simulink model "RB"  (R2024b)
settings: Solver=ode4  StartTime=0.0  StopTime=T_end_RB  FixedStep=0.01  RelTol=1e-3
values from neighbouring files (symbols this model uses):
  A = ly*lz    (= 0.25)    [Main.m]
  CD = 2.2    [Main.m]
  delta_Vz_RB = (omega_target/4)*delta_x_RB    [Main.m]
  dp0_RB = dpf_HOH    [Main.m]
  Dt = 0.01    [Main.m]
  Dt_con = 0.02    [Main.m]
  Dt_guid = 1    [Main.m]
  kf = 4    [Main.m]
  landa_RB = 1    [Main.m]
  m_c0 = 50    [Main.m]
  omega_target = (mu/r_target^3)^0.5    (= 0.00113136572666)    [Main.m]
  p0_RB = pf_HOH    [Main.m]
  rho = 1*10^(-12)    (= 1e-12)    [Main.m]
  S_RB = 0.5    [Main.m]
  T1_RB = 10    [Main.m]
  T2_RB = T1_RB + T_RB/2    (= 2786.81441073)    [Main.m]
  tau = -ton/(log(1-(Uon-Uoff)/(Tmax*kf)))    [Main.m]
  Total_max_thrust = n*Tmax    (= 2)    [Main.m]
  Uoff = 0.7    [Main.m]
  Uon = 1    [Main.m]
  Vx = omega_target*r_target    (= 7668.56094333)    [Main.m]
settings Model: Creator=corte  LastModifiedBy=aless
settings RTWCC: GPUComputeCapability=3.5

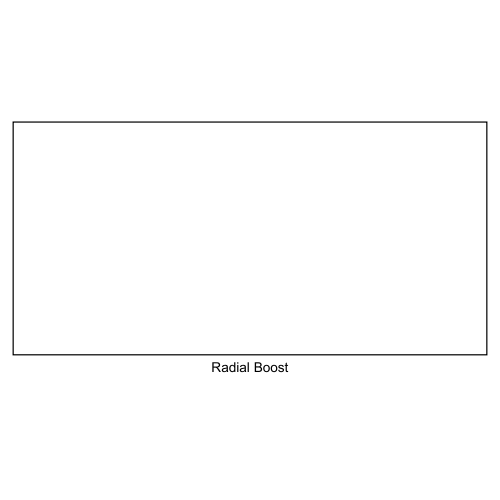
[thumbnail: Simulink's stored preview of the top-level diagram]
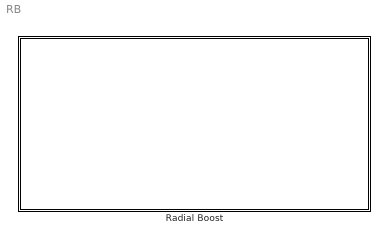
== system RB ==
  Radial Boost : Subsystem

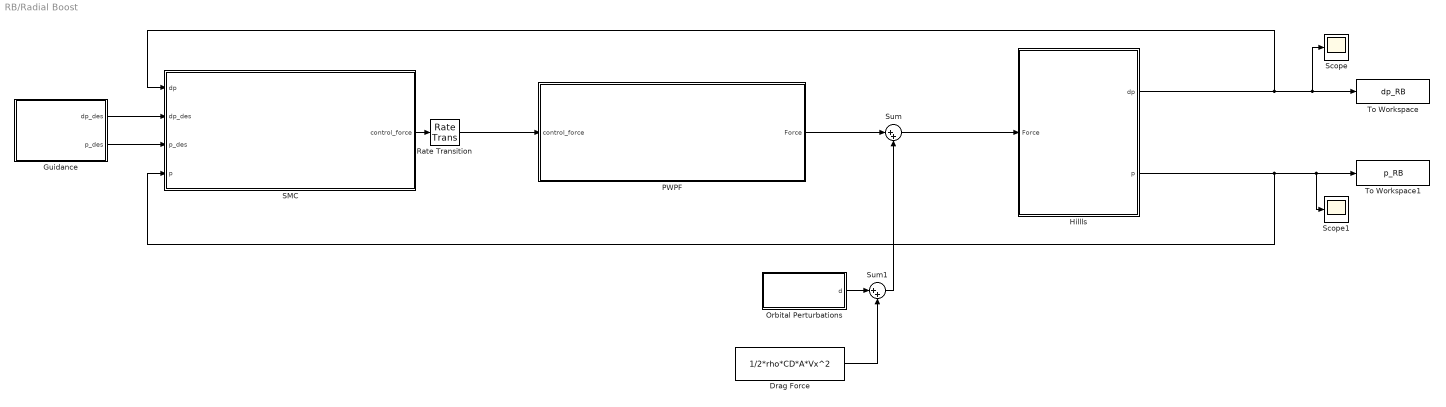
== system RB/Radial Boost ==
  Drag Force : Constant  Value=1/2*rho*CD*A*Vx^2
  Guidance : Subsystem
  Hillls : Subsystem
  Orbital Perturbations : Subsystem
  PWPF : Subsystem
  Rate Transition : RateTransition  InitialCondition=Dt_con  OutPortSampleTime=Dt
  SMC : Subsystem
  Scope : Scope
  Scope1 : Scope
  Sum : Sum  Inputs=|++
  Sum1 : Sum  Inputs=|++
  To Workspace : ToWorkspace  VariableName=dp_RB  SaveFormat=Timeseries  SampleTime=-1
  To Workspace1 : ToWorkspace  VariableName=p_RB  SaveFormat=Timeseries  SampleTime=-1
  wires:
  SMC/1(control_force) -> Rate Transition/1
  Guidance/2(p_des) -> SMC/3(p_des)
  Guidance/1(dp_des) -> SMC/2(dp_des)
  Hillls/2(p) -> Scope1/1, To Workspace1/1, SMC/4(p)
  Hillls/1(dp) -> Scope/1, To Workspace/1, SMC/1(dp)
  Rate Transition/1 -> PWPF/1(control_force)
  Sum1/1 -> Sum/2
  Drag Force/1 -> Sum1/2
  Orbital Perturbations/1(d) -> Sum1/1
  Sum/1 -> Hillls/1(Force)
  PWPF/1(Force) -> Sum/1

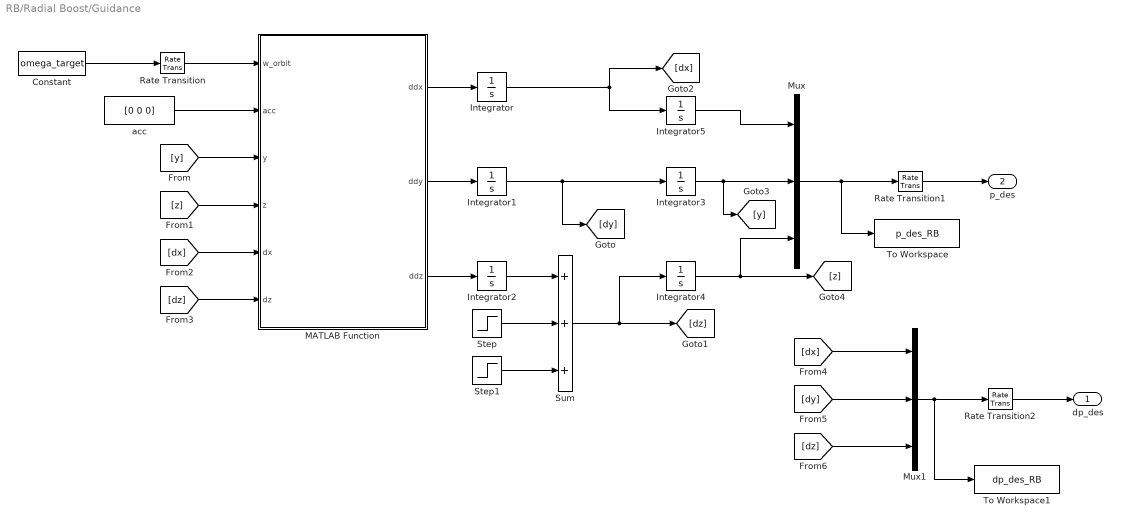
== system RB/Radial Boost/Guidance ==
  Constant : Constant  Value=omega_target
  Integrator : Integrator  InitialCondition=dp0_RB(1)
  Integrator1 : Integrator  InitialCondition=dp0_RB(2)
  Integrator2 : Integrator  InitialCondition=dp0_RB(3)
  Integrator3 : Integrator  InitialCondition=p0_RB(2)
  Integrator4 : Integrator  InitialCondition=p0_RB(3)
  Integrator5 : Integrator  InitialCondition=p0_RB(1)
  MATLAB Function : MATLAB Function  TreatAsAtomicUnit=on
  Mux : Mux  Inputs=3
  Mux1 : Mux  Inputs=3
  Rate Transition : RateTransition  InitialCondition=Dt  OutPortSampleTime=Dt_guid
  Rate Transition1 : RateTransition  InitialCondition=Dt_guid  OutPortSampleTime=Dt
  Rate Transition2 : RateTransition  InitialCondition=Dt_guid  OutPortSampleTime=Dt
  Step : Step  Time=T1_RB  After=delta_Vz_RB  SampleTime=0
  Step1 : Step  Time=T2_RB  After=delta_Vz_RB  SampleTime=0
  Sum : Sum  Inputs=+++
  To Workspace : ToWorkspace  VariableName=p_des_RB  SaveFormat=Timeseries  SampleTime=-1
  To Workspace1 : ToWorkspace  VariableName=dp_des_RB  SaveFormat=Timeseries  SampleTime=-1
  acc : Constant  Value=[0 0 0]
  dp_des : Outport
  p_des : Outport  Port=2
  wires:
  Integrator/1 -> Integrator5/1, [dx]
  Mux/1 -> Rate Transition1/1, To Workspace/1
  Integrator3/1 -> [y], Mux/2
  Integrator4/1 -> [z], Mux/3
  [y] -> MATLAB Function/3(y)
  [dx] -> Mux1/1
  [dz] -> Mux1/3
  acc/1 -> MATLAB Function/2(acc)
  MATLAB Function/1(ddx) -> Integrator/1
  Mux1/1 -> To Workspace1/1, Rate Transition2/1
  [dy] -> Mux1/2
  [dx] -> MATLAB Function/5(dx)
  [z] -> MATLAB Function/4(z)
  Integrator5/1 -> Mux/1
  Constant/1 -> Rate Transition/1
  [dz] -> MATLAB Function/6(dz)
  Integrator1/1 -> Integrator3/1, [dy]
  MATLAB Function/2(ddy) -> Integrator1/1
  Step/1 -> Sum/2
  Step1/1 -> Sum/3
  MATLAB Function/3(ddz) -> Integrator2/1
  Integrator2/1 -> Sum/1
  Sum/1 -> [dz], Integrator4/1
  Rate Transition/1 -> MATLAB Function/1(w_orbit)
  Rate Transition1/1 -> p_des/1
  Rate Transition2/1 -> dp_des/1

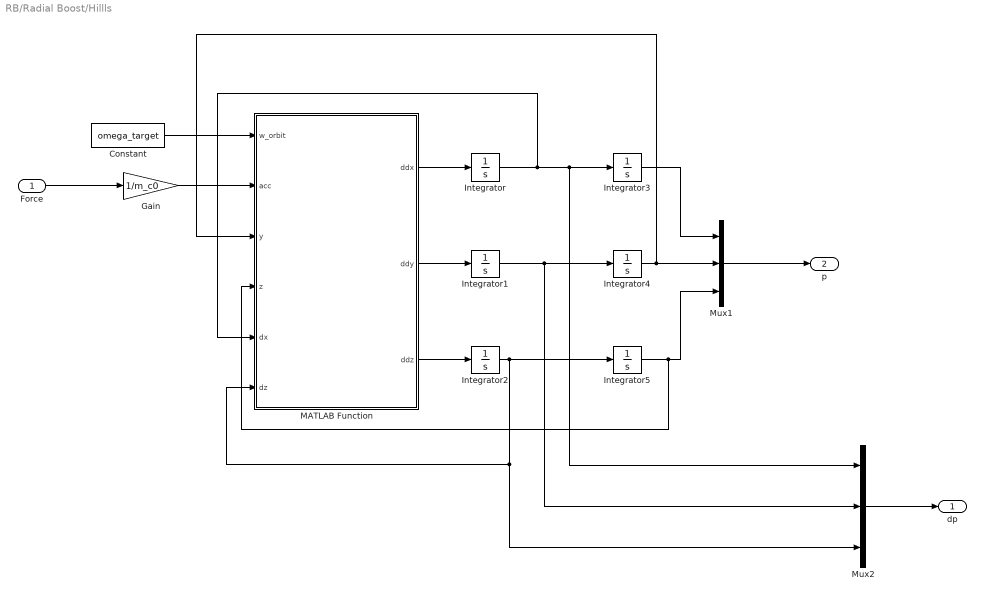
== system RB/Radial Boost/Hillls ==
  Force : Inport
  Constant : Constant  Value=omega_target
  Gain : Gain  Gain=1/m_c0
  Integrator : Integrator  InitialCondition=dp0_RB(1)
  Integrator1 : Integrator  InitialCondition=dp0_RB(2)
  Integrator2 : Integrator  InitialCondition=dp0_RB(3)
  Integrator3 : Integrator  InitialCondition=p0_RB(1)
  Integrator4 : Integrator  InitialCondition=p0_RB(2)
  Integrator5 : Integrator  InitialCondition=p0_RB(3)
  MATLAB Function : MATLAB Function  TreatAsAtomicUnit=on
  Mux1 : Mux  Inputs=3
  Mux2 : Mux  Inputs=3
  dp : Outport
  p : Outport  Port=2
  wires:
  Force/1 -> Gain/1
  Gain/1 -> MATLAB Function/2(acc)
  Constant/1 -> MATLAB Function/1(w_orbit)
  MATLAB Function/1(ddx) -> Integrator/1
  Integrator4/1 -> Mux1/2, MATLAB Function/3(y)
  Integrator3/1 -> Mux1/1
  Integrator5/1 -> Mux1/3, MATLAB Function/4(z)
  Integrator2/1 -> Integrator5/1, Mux2/3, MATLAB Function/6(dz)
  Integrator/1 -> Mux2/1, Integrator3/1, MATLAB Function/5(dx)
  MATLAB Function/2(ddy) -> Integrator1/1
  Integrator1/1 -> Mux2/2, Integrator4/1
  MATLAB Function/3(ddz) -> Integrator2/1
  Mux1/1 -> p/1
  Mux2/1 -> dp/1

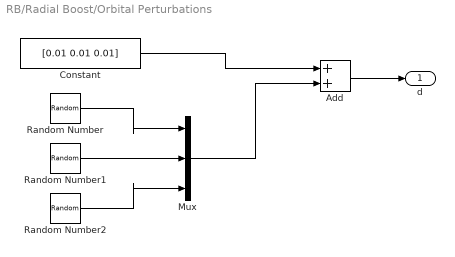
== system RB/Radial Boost/Orbital Perturbations ==
  Add : Sum
  Constant : Constant  Value=[0.01 0.01 0.01]
  Mux : Mux  Inputs=3
  Random Number : RandomNumber  Variance=(0.00001)^2  Seed=1  SampleTime=1
  Random Number1 : RandomNumber  Variance=(0.00001)^2  Seed=765  SampleTime=1
  Random Number2 : RandomNumber  Variance=(0.00001)^2  Seed=6  SampleTime=1
  d : Outport
  wires:
  Add/1 -> d/1
  Constant/1 -> Add/1
  Mux/1 -> Add/2
  Random Number2/1 -> Mux/3
  Random Number1/1 -> Mux/2
  Random Number/1 -> Mux/1

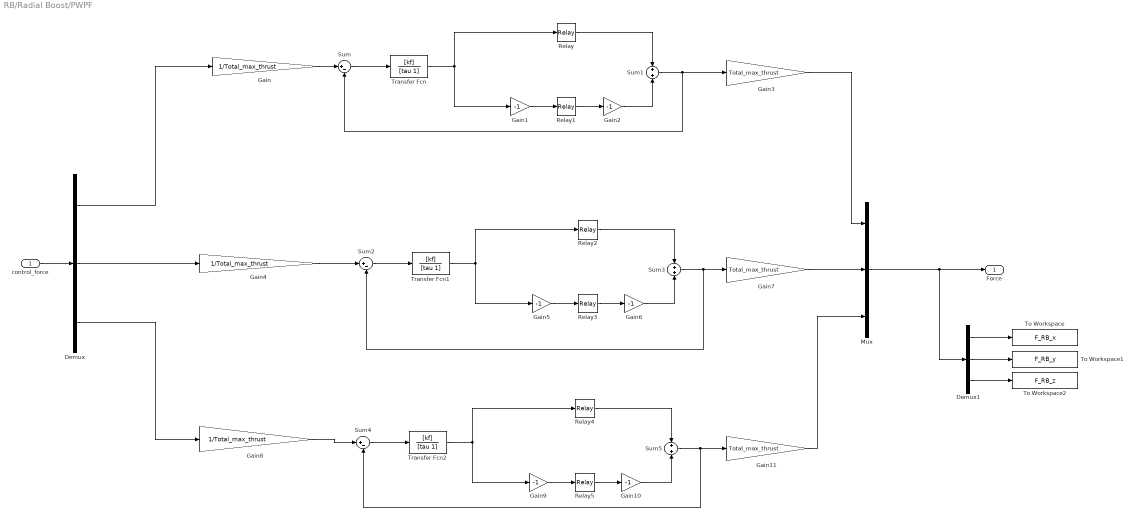
== system RB/Radial Boost/PWPF ==
  control_force : Inport
  Demux : Demux  Outputs=3
  Demux1 : Demux  Outputs=3
  Gain : Gain  Gain=1/Total_max_thrust
  Gain{1..2,5..6,9..10} (6 alike) : Gain  Gain=-1
  Gain11 : Gain  Gain=Total_max_thrust
  Gain3 : Gain  Gain=Total_max_thrust
  Gain4 : Gain  Gain=1/Total_max_thrust
  Gain7 : Gain  Gain=Total_max_thrust
  Gain8 : Gain  Gain=1/Total_max_thrust
  Mux : Mux  Inputs=3
  Relay{,1..5} (6 alike) : Relay  OnSwitchValue=Uon  OffSwitchValue=Uoff
  Sum : Sum  Inputs=|+-
  Sum1 : Sum
  Sum2 : Sum  Inputs=|+-
  Sum3 : Sum
  Sum4 : Sum  Inputs=|+-
  Sum5 : Sum
  To Workspace : ToWorkspace  VariableName=F_RB_x  SaveFormat=Timeseries  SampleTime=-1
  To Workspace1 : ToWorkspace  VariableName=F_RB_y  SaveFormat=Timeseries  SampleTime=-1
  To Workspace2 : ToWorkspace  VariableName=F_RB_z  SaveFormat=Timeseries  SampleTime=-1
  Transfer Fcn : TransferFcn  Numerator=[kf]  Denominator=[tau 1]
  Transfer Fcn1 : TransferFcn  Numerator=[kf]  Denominator=[tau 1]
  Transfer Fcn2 : TransferFcn  Numerator=[kf]  Denominator=[tau 1]
  Force : Outport
  wires:
  Gain/1 -> Sum/1
  Gain1/1 -> Relay1/1
  Relay1/1 -> Gain2/1
  Relay/1 -> Sum1/1
  Gain2/1 -> Sum1/2
  Sum1/1 -> Sum/2, Gain3/1
  Gain3/1 -> Mux/1
  Sum/1 -> Transfer Fcn/1
  Transfer Fcn/1 -> Gain1/1, Relay/1
  control_force/1 -> Demux/1
  Demux/1 -> Gain/1
  Sum3/1 -> Sum2/2, Gain7/1
  Relay3/1 -> Gain6/1
  Gain7/1 -> Mux/2
  Gain5/1 -> Relay3/1
  Relay2/1 -> Sum3/1
  Gain4/1 -> Sum2/1
  Transfer Fcn1/1 -> Gain5/1, Relay2/1
  Demux/2 -> Gain4/1
  Sum2/1 -> Transfer Fcn1/1
  Gain6/1 -> Sum3/2
  Sum5/1 -> Sum4/2, Gain11/1
  Relay5/1 -> Gain10/1
  Gain11/1 -> Mux/3
  Gain9/1 -> Relay5/1
  Relay4/1 -> Sum5/1
  Gain8/1 -> Sum4/1
  Transfer Fcn2/1 -> Gain9/1, Relay4/1
  Demux/3 -> Gain8/1
  Sum4/1 -> Transfer Fcn2/1
  Gain10/1 -> Sum5/2
  Mux/1 -> Demux1/1, Force/1
  Demux1/1 -> To Workspace/1
  Demux1/2 -> To Workspace1/1
  Demux1/3 -> To Workspace2/1

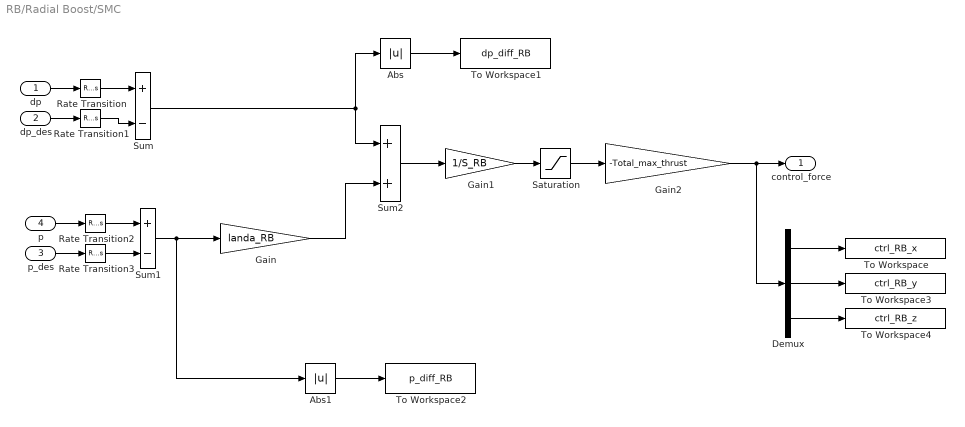
== system RB/Radial Boost/SMC ==
  dp : Inport
  dp_des : Inport  Port=2
  p_des : Inport  Port=3
  p : Inport  Port=4
  Abs : Abs  SaturateOnIntegerOverflow=off
  Abs1 : Abs  SaturateOnIntegerOverflow=off
  Demux : Demux  Outputs=3
  Gain : Gain  Gain=landa_RB
  Gain1 : Gain  Gain=1/S_RB
  Gain2 : Gain  Gain=-Total_max_thrust
  Rate Transition{,1..3} (4 alike) : RateTransition  InitialCondition=Dt  OutPortSampleTime=Dt_con
  Saturation : Saturate  UpperLimit=1  LowerLimit=-1
  Sum : Sum  Inputs=+-
  Sum1 : Sum  Inputs=+-
  Sum2 : Sum
  To Workspace : ToWorkspace  VariableName=ctrl_RB_x  SaveFormat=Timeseries  SampleTime=-1
  To Workspace1 : ToWorkspace  VariableName=dp_diff_RB  SaveFormat=Timeseries  SampleTime=-1
  To Workspace2 : ToWorkspace  VariableName=p_diff_RB  SaveFormat=Timeseries  SampleTime=-1
  To Workspace3 : ToWorkspace  VariableName=ctrl_RB_y  SaveFormat=Timeseries  SampleTime=-1
  To Workspace4 : ToWorkspace  VariableName=ctrl_RB_z  SaveFormat=Timeseries  SampleTime=-1
  control_force : Outport
  wires:
  dp/1 -> Rate Transition/1
  dp_des/1 -> Rate Transition1/1
  p/1 -> Rate Transition2/1
  p_des/1 -> Rate Transition3/1
  Sum1/1 -> Abs1/1, Gain/1
  Gain/1 -> Sum2/2
  Sum/1 -> Abs/1, Sum2/1
  Sum2/1 -> Gain1/1
  Gain1/1 -> Saturation/1
  Saturation/1 -> Gain2/1
  Gain2/1 -> control_force/1, Demux/1
  Abs/1 -> To Workspace1/1
  Abs1/1 -> To Workspace2/1
  Rate Transition/1 -> Sum/1
  Rate Transition1/1 -> Sum/2
  Rate Transition2/1 -> Sum1/1
  Rate Transition3/1 -> Sum1/2
  Demux/1 -> To Workspace/1
  Demux/2 -> To Workspace3/1
  Demux/3 -> To Workspace4/1

== matlab function RB/Radial Boost/Hillls/MATLAB Function ==
  data: w_orbit input; ddx output size=1; acc input; y input; z input; dx input; dz input; ddy output size=1; ddz output size=1
function [ddx, ddy, ddz] = fcn(w_orbit, acc, y, z, dx, dz)
ddx=acc(1)+2*w_orbit*dz;
ddy=acc(2)+w_orbit^2*y;
ddz=acc(3)+3*w_orbit^2*z-2*w_orbit*dx;

end

== matlab function RB/Radial Boost/Guidance/MATLAB Function ==
  data: w_orbit input; ddx output; acc input; y input; z input; dx input; dz input; ddy output; ddz output
function [ddx, ddy, ddz] = fcn(w_orbit, acc, y, z, dx, dz)
ddx=acc(1)+2*w_orbit*dz;
ddy=acc(2)+w_orbit^2*y;
ddz=acc(3)+3*w_orbit^2*z-2*w_orbit*dx;

end
